simulink model "inputOutputControl"  (R2023b)
settings: Solver=VariableStepAuto  StartTime=0.0  StopTime=t(end)  RelTol=1e-3
values from neighbouring files (symbols this model uses):
  b = 0.2    [pathPlanning.m]
libraries: robotmobilelib x1
settings Model: Creator=v4pal  LastModifiedBy=v4pal

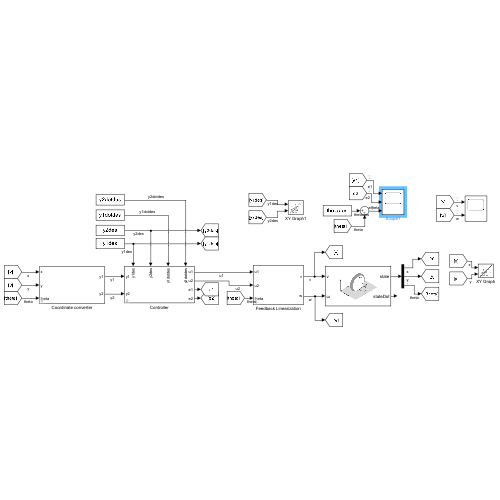
[thumbnail: Simulink's stored preview of the top-level diagram]
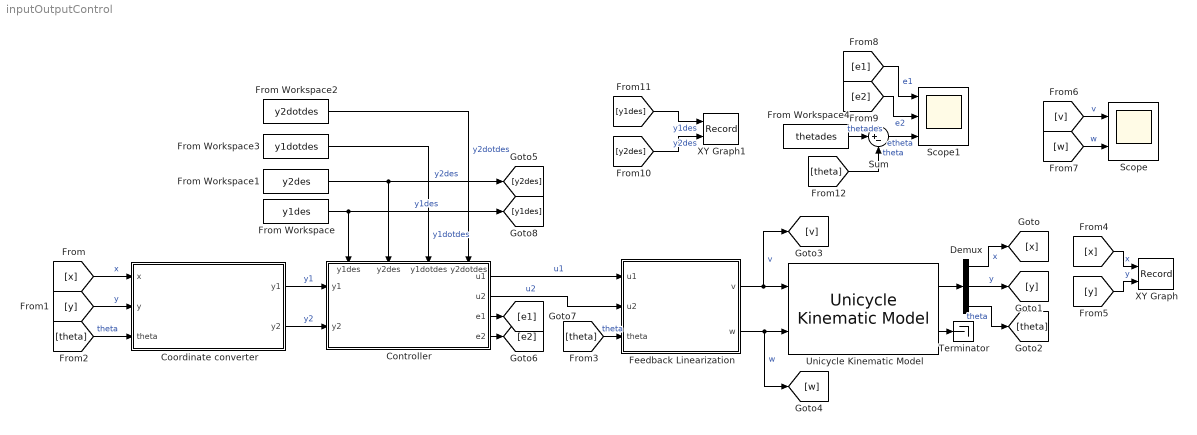
== system inputOutputControl ==
  Controller : Subsystem  mask{k1=5, k2=5}
      settings: PortSchema="{\"entries\":[{\"content\":{\"sides\":[{\"content\":{\"connectorIds\":[\"In1\",\"In2\"]},\"type\":\"ConnectorPlacement.EquallySpacedRectSide\",\"uuid\":\"3a3a90f3-9643-4557-adb2-38e9acf145b1\"},{\"content\":{\"connectorIds\":[\"Out1\",\"Out2\",\"Out3\",\"Out4\"],\"side\":\"RIGHT\"},\"type\":\"ConnectorPlacement.EquallySpacedRectSide\",\"uuid\":\"b4861c96-dfb4-40fc-837d-ca342de7e81f\"},{\"content\":{\"connectorIds\":[\"In3\",\"In4\",\"In5\",\"In6\"],\"side\":\"TOP\"},\"type\":\"ConnectorPlacement.EquallySpacedRectSide\",\"uuid\":\"e9f8ee6b-112e-4c13-8ae8-8c12efb828c1\"}]},\"type\":\"ConnectorPlacement.EquallySpacedConnector\",\"uuid\":\"1b64a635-0329-4f5b-ba47-74872ea41b94\"}],\"packageUris\":[\"http://schema.mathworks.com/mf0/Connector/R2020b\"],\"version\":\"1.0\"}"
  Coordinate converter : Subsystem  mask{b=b}
  Demux : Demux  Outputs=3
  Feedback Linearization : Subsystem  mask{b=b}
  From Workspace : FromWorkspace  VariableName=y1des
  From Workspace1 : FromWorkspace  VariableName=y2des
  From Workspace2 : FromWorkspace  VariableName=y2dotdes
  From Workspace3 : FromWorkspace  VariableName=y1dotdes
  From Workspace4 : FromWorkspace  VariableName=thetades
  Scope : Scope  NumInputPorts=2
  Scope1 : Scope  NumInputPorts=3
  Sum : Sum  Inputs=|+-
  Terminator : Terminator
  Unicycle Kinematic Model : robotmobilelib/Unicycle Kinematic Model  VehicleInputs=Vehicle Speed & Heading Angular Velocity  WheelRadius=0.1  WheelSpeedRange=[-Inf Inf]  InitialState=qi  SimulateUsing=Interpreted execution
  XY Graph : Record  FileSettingsInternal="{\"entries\":[{\"content\":{\"excelSettings\":{\"content\":{},\"type\":\"Streamout.ExcelSettings\"}},\"type\":\"Streamout.FileSettingStorage\",\"uuid\":\"\"}],\"packageUris\":[\"http:\\/\\/schema.mathworks.com\\/mf0\\/streamout_blocks\\/R2020a\"],\"version\":\"1.0\"}"  Layout=[1 1]  SignalsInternal="{\"entries\":[{\"content\":{\"signals\":[{\"content\":{\"blockPath\":[],\"dimensions\":[1],\"domain\":\"\",\"lineColor\":\"#64d413\",\"port\":1,\"sid\":[\"\"],\"signalID\":1218,\"signalName\":\"x\"},\"type\":\"RecordBlkView.Signal\",\"uuid\":\"\"},{\"content\":{\"blockPath\":[],\"dimensions\":[1],\"domain\":\"\",\"lineColor\":\"#ff13a6\",\"port\":2,\"sid\":[\"\"],\"signalID\":1222,\"signalName\":\"y\"},\"type\":\"RecordBlkView.Signal\",\"uuid\":\"\"}]},\"type\":\"RecordBlkView.InputSignals\",\"uuid\":\"\"}],\"packageUris\":[\"http:\\/\\/schema.mathworks.com\\/mf0\\/streamout_blocks\\/R2020a\"],\"version\":\"1.0\"}"  VisualizationBindings="{\"xyplotplugin\":{\"info\":[{\"series\":[{\"bindingParametersList\":[{\"parameter\":\"X-Axis\",\"signalID\":1029,\"signalName\":\"x\"},{\"parameter\":\"Y-Axis\",\"signalID\":1033,\"signalName\":\"y\"}],\"seriesID\":50595}],\"subplotID\":1}]}}"  CompatibilityTag=XY
  XY Graph1 : Record  FileSettingsInternal="{\"entries\":[{\"content\":{\"excelSettings\":{\"content\":{},\"type\":\"Streamout.ExcelSettings\"}},\"type\":\"Streamout.FileSettingStorage\",\"uuid\":\"\"}],\"packageUris\":[\"http:\\/\\/schema.mathworks.com\\/mf0\\/streamout_blocks\\/R2020a\"],\"version\":\"1.0\"}"  Layout=[1 1]  SignalsInternal="{\"entries\":[{\"content\":{\"signals\":[{\"content\":{\"blockPath\":[],\"dimensions\":[1],\"domain\":\"\",\"lineColor\":\"#fe330a\",\"port\":1,\"sid\":[\"\"],\"signalID\":1226,\"signalName\":\"y1des\"},\"type\":\"RecordBlkView.Signal\",\"uuid\":\"\"},{\"content\":{\"blockPath\":[],\"dimensions\":[1],\"domain\":\"\",\"lineColor\":\"#22b573\",\"port\":2,\"sid\":[\"\"],\"signalID\":1230,\"signalName\":\"y2des\"},\"type\":\"RecordBlkView.Signal\",\"uuid\":\"\"}]},\"type\":\"RecordBlkView.InputSignals\",\"uuid\":\"\"}],\"packageUris\":[\"http:\\/\\/schema.mathworks.com\\/mf0\\/streamout_blocks\\/R2020a\"],\"version\":\"1.0\"}"  VisualizationBindings="{\"xyplotplugin\":{\"info\":[{\"series\":[{\"bindingParametersList\":[{\"parameter\":\"X-Axis\",\"signalID\":1037,\"signalName\":\"y1des\"},{\"parameter\":\"Y-Axis\",\"signalID\":1041,\"signalName\":\"y2des\"}],\"seriesID\":32925}],\"subplotID\":1}]}}"  CompatibilityTag=XY
  wires:
  Unicycle Kinematic Model/1 -> Demux/1
  Demux/3 -> [theta]  "theta"
  Demux/1 -> [x]  "x"
  Demux/2 -> [y]  "y"
  Feedback Linearization/1(v) -> [v], Unicycle Kinematic Model/1  "v"
  Feedback Linearization/2(w) -> [w], Unicycle Kinematic Model/2  "w"
  From Workspace1/1 -> [y2des], Controller/4(y2des)  "y2des"
  From Workspace2/1 -> Controller/6(y2dotdes)  "y2dotdes"
  From Workspace/1 -> [y1des], Controller/3(y1des)  "y1des"
  From Workspace3/1 -> Controller/5(y1dotdes)  "y1dotdes"
  Coordinate converter/1(y1) -> Controller/1(y1)  "y1"
  Coordinate converter/2(y2) -> Controller/2(y2)  "y2"
  Controller/1(u1) -> Feedback Linearization/1(u1)  "u1"
  Controller/2(u2) -> Feedback Linearization/2(u2)  "u2"
  Unicycle Kinematic Model/2 -> Terminator/1
  [x] -> Coordinate converter/1(x)  "x"
  [y] -> Coordinate converter/2(y)  "y"
  [theta] -> Coordinate converter/3(theta)  "theta"
  [theta] -> Feedback Linearization/3(theta)  "theta"
  [x] -> XY Graph/1  "x"
  [y] -> XY Graph/2  "y"
  [v] -> Scope/1  "v"
  [w] -> Scope/2  "w"
  Controller/3(e1) -> [e1]
  Controller/4(e2) -> [e2]
  [e1] -> Scope1/1  "e1"
  [e2] -> Scope1/2  "e2"
  [y1des] -> XY Graph1/1  "y1des"
  [y2des] -> XY Graph1/2  "y2des"
  From Workspace4/1 -> Sum/1  "thetades"
  [theta] -> Sum/2  "theta"
  Sum/1 -> Scope1/3  "etheta"

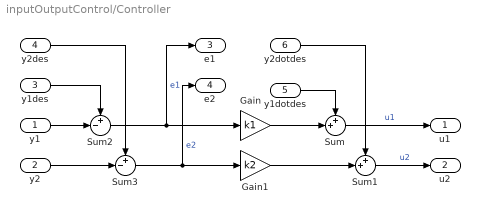
== system inputOutputControl/Controller ==
  y1 : Inport
  y2 : Inport  Port=2
  y1des : Inport  Port=3
  y2des : Inport  Port=4
  y1dotdes : Inport  Port=5
  y2dotdes : Inport  Port=6
  Gain : Gain  Gain=k1
  Gain1 : Gain  Gain=k2
  Sum : Sum  Inputs=++|
  Sum1 : Sum  Inputs=++|
  Sum2 : Sum  Inputs=+-|
  Sum3 : Sum  Inputs=+-|
  u1 : Outport
  u2 : Outport  Port=2
  e1 : Outport  Port=3
  e2 : Outport  Port=4
  wires:
  Sum1/1 -> u2/1  "u2"
  Sum2/1 -> e1/1, Gain/1  "e1"
  y2dotdes/1 -> Sum1/1
  Gain1/1 -> Sum1/2
  y1/1 -> Sum2/2
  y2/1 -> Sum3/2
  Gain/1 -> Sum/2
  Sum/1 -> u1/1  "u1"
  Sum3/1 -> e2/1, Gain1/1  "e2"
  y2des/1 -> Sum3/1
  y1des/1 -> Sum2/1
  y1dotdes/1 -> Sum/1

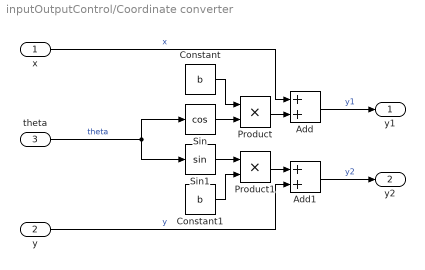
== system inputOutputControl/Coordinate converter ==
  x : Inport
  y : Inport  Port=2
  theta : Inport  Port=3
  Add : Sum
  Add1 : Sum
  Constant : Constant  Value=b
  Constant1 : Constant  Value=b
  Product : Product
  Product1 : Product
  Sin : Trigonometry  Operator=cos
  Sin1 : Trigonometry
  y1 : Outport
  y2 : Outport  Port=2
  wires:
  Sin1/1 -> Product1/1
  Product/1 -> Add/2
  theta/1 -> Sin/1, Sin1/1  "theta"
  Add1/1 -> y2/1  "y2"
  Constant1/1 -> Product1/2
  Sin/1 -> Product/2
  Product1/1 -> Add1/1
  x/1 -> Add/1  "x"
  Constant/1 -> Product/1
  y/1 -> Add1/2  "y"
  Add/1 -> y1/1  "y1"

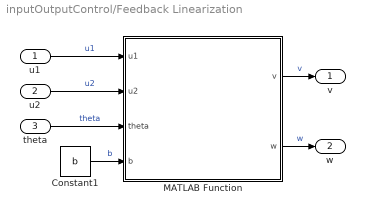
== system inputOutputControl/Feedback Linearization ==
  u1 : Inport
  u2 : Inport  Port=2
  theta : Inport  Port=3
  Constant1 : Constant  Value=b
  MATLAB Function : MATLAB Function  TreatAsAtomicUnit=on
  v : Outport
  w : Outport  Port=2
  wires:
  Constant1/1 -> MATLAB Function/4(b)  "b"
  theta/1 -> MATLAB Function/3(theta)  "theta"
  u1/1 -> MATLAB Function/1(u1)  "u1"
  MATLAB Function/1(v) -> v/1  "v"
  MATLAB Function/2(w) -> w/1  "w"
  u2/1 -> MATLAB Function/2(u2)  "u2"

== matlab function inputOutputControl/Feedback Linearization/MATLAB Function ==
  data: u1 input; v output; u2 input; theta input; b input; w output
function [v, w] = Tinv(u1, u2, theta, b)

    T = [cos(theta), -b*sin(theta);
        sin(theta), b*cos(theta);];

    invT = T^-1;

    v = invT(1,1) * u1 + invT(1,2) * u2;
    w = invT(2,1) * u1 + invT(2,2) * u2;
